simulink model "q2_partcpartd"  (R2018b)
settings: Solver=VariableStepAuto  StartTime=0.0  StopTime=30  RelTol=1e-3
settings Model: Creator=Ahmet Asım  LastModifiedBy=Ahmet Asım

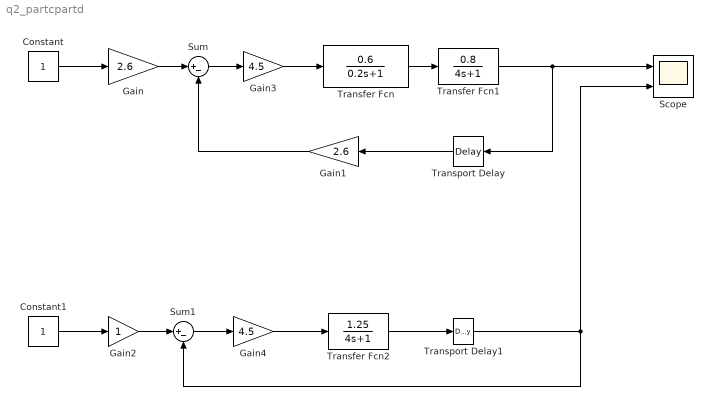
== system q2_partcpartd ==
  Constant : Constant
  Constant1 : Constant
  Gain : Gain  Gain=2.6
  Gain1 : Gain  Gain=2.6
  Gain2 : Gain
  Gain3 : Gain  Gain=4.5
  Gain4 : Gain  Gain=4.5
  Scope : Scope  NumInputPorts=2
  Sum : Sum  Inputs=|+-
  Sum1 : Sum  Inputs=|+-
  Transfer Fcn : TransferFcn  Numerator=[0.6]  Denominator=[0.2 1]
  Transfer Fcn1 : TransferFcn  Numerator=[0.8]  Denominator=[4 1]
  Transfer Fcn2 : TransferFcn  Numerator=[1.25]  Denominator=[4 1]
  Transport Delay : TransportDelay  DelayTime=0.725
  Transport Delay1 : TransportDelay  DelayTime=0.925
  wires:
  Gain4/1 -> Transfer Fcn2/1
  Constant/1 -> Gain/1
  Constant1/1 -> Gain2/1
  Sum/1 -> Gain3/1
  Gain3/1 -> Transfer Fcn/1
  Transfer Fcn/1 -> Transfer Fcn1/1
  Transport Delay/1 -> Gain1/1
  Transport Delay1/1 -> Scope/2, Sum1/2
  Gain/1 -> Sum/1
  Gain2/1 -> Sum1/1
  Transfer Fcn1/1 -> Transport Delay/1, Scope/1
  Gain1/1 -> Sum/2
  Transfer Fcn2/1 -> Transport Delay1/1
  Sum1/1 -> Gain4/1
